simulink model "sistema_control"  (Simulink 7.9)
settings: Solver=ode45  StartTime=0.0  StopTime=Tt  RelTol=1e-3
undefined symbols (not defined in the file): a, A, Ad, b, B, Bd, c, C, Cd, D, Dd, K, Kc, Kd, r, Ts, x1, x2, x3, x4
libraries: simulink x1
settings Model: Creator=pdoren  LastModifiedBy=pdoren  CovModelRefEnable=off
settings DataIOCC: SaveFormat=StructureWithTime  SignalLoggingSaveFormat=Dataset
settings OptimizationCC: ExpressionDepthLimit=128
settings DebuggingCC: UnderspecifiedInitializationDetection=Simplified  MergeDetectMultiDrivingBlocksExec=error  SolverPrmCheckMsg=none  FrameProcessingCompatibilityMsg=error  StateNameClashWarn=none
settings HardwareCC: ProdBitPerPointer=64  ProdLargestAtomicFloat=Float  ProdIntDivRoundTo=Zero  ProdEndianess=LittleEndian  ProdHWDeviceType=Specified
settings CodeAppCC: CustomSymbolStrType=$N$R$M_T
settings GRTTargetCC: CodeReplacementLibrary=C89/C90 (ANSI)  GeneratePreprocessorConditionals=Use local settings

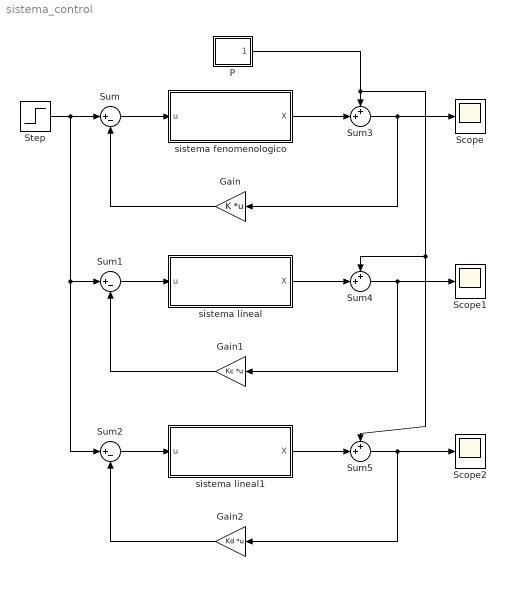
== system sistema_control ==
  Gain : Gain  Gain=K  Multiplication=Matrix(K*u)
  Gain1 : Gain  Gain=Kc  Multiplication=Matrix(K*u)
  Gain2 : Gain  Gain=Kd  Multiplication=Matrix(K*u)
  P : Subsystem
  Scope : Scope
      settings: TimeRange=auto  MaxDataPoints=5000  SaveName=estados_fenomenologico  YMin=-0.0879  YMax=0.09213  SampleTime=-1  DataFormat=Array
  Scope1 : Scope
      settings: TimeRange=auto  MaxDataPoints=5000  SaveName=estados_lineal  YMin=-139451949409836570000000000000.00000  YMax=1255067544688529400000000000000.00000  SampleTime=-1  DataFormat=Array
  Scope2 : Scope
      settings: TimeRange=auto  MaxDataPoints=5000  SaveName=estados_lineal_discreto  YMin=-39.31705  YMax=355.85342  SampleTime=-1  DataFormat=Array
  Step : Step  After=r  SampleTime=0
  Sum : Sum  Inputs=|+-
  Sum1 : Sum  Inputs=|+-
  Sum2 : Sum  Inputs=|+-
  Sum3 : Sum  Inputs=++|
  Sum4 : Sum  Inputs=++|
  Sum5 : Sum  Inputs=++|
  sistema fenomenologico : Subsystem
  sistema lineal : Subsystem
  sistema lineal1 : Subsystem
  wires:
  Sum/1 -> sistema fenomenologico/1(u)
  Step/1 -> Sum2/1, Sum1/1, Sum/1
  Gain/1 -> Sum/2
  Sum1/1 -> sistema lineal/1(u)
  Sum2/1 -> sistema lineal1/1(u)
  Gain1/1 -> Sum1/2
  Gain2/1 -> Sum2/2
  sistema fenomenologico/1(X) -> Sum3/2
  Sum3/1 -> Gain/1, Scope/1
  sistema lineal/1(X) -> Sum4/2
  Sum4/1 -> Gain1/1, Scope1/1
  sistema lineal1/1(X) -> Sum5/2
  Sum5/1 -> Gain2/1, Scope2/1
  P/1(Out1) -> Sum5/1, Sum4/1, Sum3/1

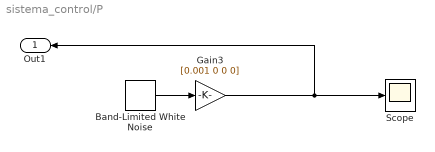
== system sistema_control/P ==
  Band-Limited White Noise : simulink/Sources/Band-Limited White Noise  Cov=[0.01]  Ts=0.002  seed=[23341]
  Gain3 : Gain  Gain=[0.001 0 0 0]
  Scope : Scope
      settings: TimeRange=auto  MaxDataPoints=5000  SaveToWorkspace=off  YMin=-0.01017  YMax=0.01093  SampleTime=-1
  Out1 : Outport
  wires:
  Gain3/1 -> Out1/1, Scope/1
  Band-Limited White Noise/1 -> Gain3/1

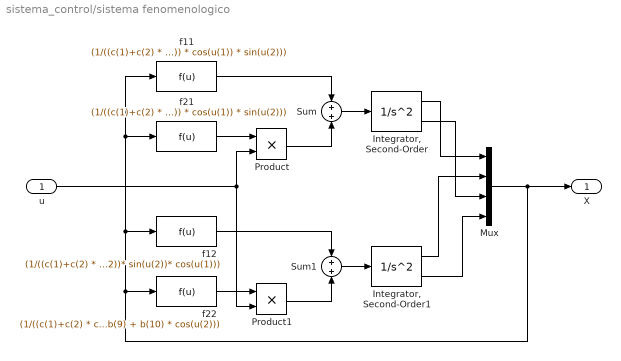
== system sistema_control/sistema fenomenologico ==
  u : Inport
  "Integrator, Second-Order" : SecondOrderIntegrator  ICX=x1  ICDXDT=x3
  "Integrator, Second-Order1" : SecondOrderIntegrator  ICX=x2  ICDXDT=x4
  Mux : Mux
  Product : Product
  Product1 : Product
  Sum : Sum  Inputs=+|+
  Sum1 : Sum  Inputs=+|+
  f11 : Fcn  Expr=(1/((c(1)+c(2) * cos(u(2))^2) * c(3))) * ((a(1) + a(2) * cos(u(2))) * sin(u(2)) * u(3)^2 + a(3) * sin(u(2)) * u(4) * u(3) + a(4) * sin(u(2)) * u(4)^2 + (a(5) + a(6) * cos(u(2))) * u(4) + a(9) * sin(u(1)) * cos(u(2))^2 + a(10) * sin(u(1)) + a(11) * cos(u(2)) * cos(u(1)) * sin(u(2)))
  f12 : Fcn  Expr=(1/((c(1)+c(2) * cos(u(2))^2) * c(3))) * ((b(1) + b(2) * cos(u(2))) * sin(u(2)) * u(3)^2 + (b(3) * cos(u(2)) + b(4))* sin(u(2)) * u(4) * u(1) + (b(5) + b(6) * cos(u(2)))* sin(u(2)) * u(4)^2 + (b(7) + b(8)* cos(u(2))) * u(4) + (b(11) + b(12)* cos(u(2)))* sin(u(1)) + b(13) * sin(u(1)) * cos(u(2))^2 + b(14) * cos(u(1)) * sin(u(2)) + b(15) * cos(u(2))* sin(u(2))* cos(u(1)))
  f21 : Fcn  Expr=(1/((c(1)+c(2) * cos(u(2))^2) * c(3))) * ((a(1) + a(2) * cos(u(2))) * sin(u(2)) * u(3)^2 + a(3) * sin(u(2)) * u(4) * u(3) + a(4) * sin(u(2)) * u(4)^2 + (a(5) + a(6) * cos(u(2))) * u(4) + a(9) * sin(u(1)) * cos(u(2))^2 + a(10) * sin(u(1)) + a(11) * cos(u(2)) * cos(u(1)) * sin(u(2)))
  f22 : Fcn  Expr=(1/((c(1)+c(2) * cos(u(2))^2) * c(3))) * (b(9) + b(10) * cos(u(2)))
  X : Outport
  wires:
  Product/1 -> Sum/2
  f11/1 -> Sum/1
  f21/1 -> Product/1
  "Integrator, Second-Order"/1 -> Mux/1
  "Integrator, Second-Order1"/2 -> Mux/4
  Sum1/1 -> "Integrator, Second-Order1"/1
  "Integrator, Second-Order"/2 -> Mux/3
  "Integrator, Second-Order1"/1 -> Mux/2
  u/1 -> Product1/2, Product/2
  Mux/1 -> X/1, f22/1, f12/1, f21/1, f11/1
  Sum/1 -> "Integrator, Second-Order"/1
  f12/1 -> Sum1/1
  f22/1 -> Product1/1
  Product1/1 -> Sum1/2

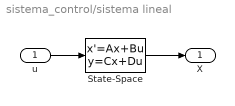
== system sistema_control/sistema lineal ==
  u : Inport
  State-Space : StateSpace  A=A  B=B  C=C  D=D  X0=[x1 x2 x3 x4]
  X : Outport
  wires:
  u/1 -> State-Space/1
  State-Space/1 -> X/1

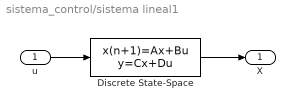
== system sistema_control/sistema lineal1 ==
  u : Inport
  Discrete State-Space : DiscreteStateSpace  A=Ad  B=Bd  C=Cd  D=Dd  X0=[x1 x2 x3 x4]  SampleTime=Ts
  X : Outport
  wires:
  u/1 -> Discrete State-Space/1
  Discrete State-Space/1 -> X/1
